simulink model "backbone"  (R2022b)
settings: Solver=FixedStepDiscrete  StartTime=0.0  StopTime=2  FixedStep=0.000001  RelTol=1e-3
undefined symbols (not defined in the file or in its folder): DiscIntNeverNeededParam, flux, Motor_flux, Motor_Ld_Indctances, Motor_Lq_Indctances, Motor_Pn, Motor_Rs, Pn, switch_electronic_feedworward, Switch_SubsysCtrl, SysCurrentMax, SysVoltage, Ts
libraries: powerlib_extras x11, simulink x4, mcbcontrolslib x4, slpidlib x3, spsPermanentMagnetSynchronousMachineLib x2, spsDCVoltageSourceLib x2, spsGroundLib x1, eePmsmCurrentController x1, spsThreePhaseVIMeasurementLib x1, spsTwoLevelConverterLib x1, spsUniversalBridgeLib x1, spspowerguiLib x1
(part 3 of 3)

== matlab function backbone/Variant Subsystem/MPTA_MPTV_PMSM/MPTA_弱磁/MPTA_MPTV_Base_IMax /MPTA_MPTV_Imax ==
  data: iqPIDref input; idref output; iqref output; UI input; LdLqPnFluxRs input; state output; clock input; we input; last_state input; We_A output; We_B output; Zone output; ctrl_way2 output; Te output
function [idref, iqref,state,We_A,We_B,Zone,ctrl_way2,Te] = fcn(iqPIDref, UI, LdLqPnFluxRs, clock, we, last_state)

% https://blog.csdn.net/weixin_44312889/article/details/124467496
%%%%%%%%%%%%%%%%%%%%%%%%%%%%%%%%%%%%%
%               读取数据
Udc=UI(1);
I=UI(2);
Ld=LdLqPnFluxRs(1);
Lq=LdLqPnFluxRs(2);
pn=LdLqPnFluxRs(3);%转子对数
flux=LdLqPnFluxRs(4);%永磁体磁链
R=LdLqPnFluxRs(5); %定子电阻
Zone=0;
ctrl_way2=0;

Umax=Udc/sqrt(3); %最大电压限制 此处应该是相电压最大值 
Imax=I*sqrt(2);% 最大电流限制

%%%%%%%%%%%%%%%%%%%%%%%%%%%%%%%%%%%%%
%               计算最大电流下MPTA与最大电流圆的交点A
IdA=(-flux+sqrt(flux^2+8*(Ld-Lq)^2*Imax^2))/(4*(Ld-Lq));
IqA=sqrt(Imax^2 - IdA^2);
We_A=sqrt(Umax^2/((Ld*IdA+flux)^2+(Lq*IqA)^2));
ctrl_way2=IqA;

%               计算最大电流下MPTV与最大电压圆的交点B
a=4*(Ld-Lq)^2*Ld^2+4*Lq^2*(Ld-Lq)^2;
b=8*flux*Ld*(Ld-Lq)^2+4*flux*Lq*(Ld-Lq)*Ld;
c=4*flux^2*(Ld-Lq)^2+4*flux^2*Lq*(Ld-Lq)-4*Lq^2*(Ld-Lq)^2*Imax^2;
IdB=(-b-sqrt(b^2-4*a*c))/(2*a);
tempB_a=-flux*Ld*(2*Ld-Lq);
tempB_b=2*(Ld^2+Lq^2)*(Ld-Lq);
tempB_c=Ld^2*(2*Ld-Lq)^2-4*Ld*(Ld-Lq)*(Ld^2+Lq^2);
tempB_d=Lq^2*(Ld-Lq)^2*(Ld^2+Lq^2);
tempB_e=sqrt(tempB_c*flux^2+4*Imax^2*tempB_d);

IdB=tempB_a+tempB_e/tempB_b;
IqB=sqrt(Imax^2-IdB^2);


We_B=sqrt(Umax^2/((Ld*IdB+flux)^2+(Lq*IqB)^2));
state=0;


% 进行MPTA控制 
iqref = iqPIDref;                           
idref=-flux+sqrt(flux^2+4*(Ld-Lq)^2*iqref^2)/(2*(Ld-Lq));

if(we<=We_A)
    if(iqPIDref<IqA) 
        % MPTA控制
        iqref = iqPIDref; % 此时进行MPTA控制   如果 iqref∈(-IqA,IqA)之间 则通过MPTA曲线上的idref
        idref=-flux+sqrt(flux^2+4*(Ld-Lq)^2*iqref^2)/(2*(Ld-Lq)); 
        Zone=0;
    else
        % 此时已达最大
        iqref=IqA;
        idref=IdA;
        Zone=1;
    end
elseif(we>We_A&&we<We_B)
       % FW iq id 沿着极限电压圆的轨迹变换
        idAB =(-flux*Ld+sqrt(flux^2*Ld^2-(Ld^2-Lq^2)*(flux^2+Lq^2*Imax^2-(Umax/we)^2)))/(Ld^2-Lq^2);
        iqAB =sqrt(Imax^2 - idAB^2);
        if(iqPIDref<iqAB)
            %idref=(-flux*Ld+sqrt(flux^2*Ld^2-(Ld^2-Lq^2)*(flux^2+Lq^2*iqPIDref^2-(Umax/we)^2)))/(Ld^2-Lq^2);
            temp=flux^2*Ld^2-(Ld^2-Lq^2)*(flux^2+Lq^2*iqPIDref^2-(Umax/we)^2); 
            idref=-(-flux*Ld+real(sqrt(complex(temp))))/(Ld^2-Lq^2);% 感觉我这步有点问题
            iqref=iqPIDref;
            Zone=2;
        else
            idref=idAB;
            iqref=iqAB;
            Zone=3;
        end
else %we > we_B MPTV
        idMTPV=-flux/Ld+(-flux*Lq+sqrt(flux^2*Lq^2+8*(Ld-Lq)^2*(Umax/we)^2))/(4*Ld*(Ld-Lq));
        iqMTPV=sqrt((Umax^2/we^2 - (Ld*idMTPV*flux)^2)/Lq^2); 
        if(iqPIDref<iqMTPV)
            iqref=iqPIDref;             
            idref=-flux/Ld+(-flux*Lq+Lq*sqrt(flux^2+4*(Ld-Lq)^2*iqref^2))/(2*Ld*(Ld-Lq));
            Zone=4;
        else
            idref=idMTPV;
            iqref=iqMTPV;
            Zone=5;
        end
end

        Te=3/2*pn*(flux*iqref+(Ld-Lq)*idref*iqref);
end

== matlab function backbone/Variant Subsystem/MPTA_MPTV_PMSM/MPTA_弱磁/MPTA_MPTV_Base_Te/MPTA_MPTV_Imax ==
  data: wx input; iqref_raw input; idref output; iqref output; UI input; LdLqPnFluxRs input; we input
function [idref, iqref] = fcn(wx,iqref_raw, UI, LdLqPnFluxRs, we)


%%%%%%%%%%%%%%%%%%%%%%%%%%%%%%%%%%%%%
%               读取数据


Udc=UI(1);
I=UI(2);
Ld=LdLqPnFluxRs(1);
Lq=LdLqPnFluxRs(2);
pn=LdLqPnFluxRs(3);
flux=LdLqPnFluxRs(4);
R=LdLqPnFluxRs(5);
psif=flux;

Umax=Udc*2/pi;
Imax=I*sqrt(2);

%%%%%%%%%%%%%%%%%%%%%%%%%%%%%%%%%%%%%

% id=0;
% iq=0;
p=Lq/Ld;%凸极率
num = flux^2+8*(Ld-Lq)^2*Ilim^2;
C = -flux+sqrt(num);
num0 = (Lq*Ilim)^2+flux^2+((Ld+Lq)*C^2+8*flux*Ld*C)/(16*(Ld-Lq));
nb = 60*Ulim/(2*pi*sqrt(num0));
wb = Pn*nb*pi/30;%基速 电角速度
% id、iq是电流环的给定，也就是MTPA的输出，无法用星号表示
% MPTA相关
    num1 = 8*Te*flux/(3*Pn);
    num2 = flux^2-4*(Ld-Lq)^2;
    num4 = num1^2-4*num2*((0.5*num1/flux)^2-flux^2);
    
    num3 = flux*0.5/(Lq-Ld);
    
    
if(wx<=wb)                % MPTA
    % 第一步 计算iq
    iq = (num1+sqrt(num4))/(2*num2);
 
    %第二步 计算id
    num5 = 0.25*flux^2/(Ld-Lq)^2+iq^2;
    id = num3-sqrt(num5);
else                      %弱磁控制
    if(we<wx)      %到达C点之前       
        if(flux/Ld>Ilim)
            num6 = flux^2*Ld^2-(Ld^2-Lq^2)*(flux^2-Ulim^2/wx^2+Lq^2*Ilim^2);
            id = (-flux*Ld+sqrt(num6))/(Ld^2-Lq^2);
            num7 = Ilim^2-id^2;
            iq = sqrt(num7); %显 示7为负
        else
            num8 = flux^2*Ld^2-(Lq^2-Ld^2)*(Ulim^2/wx^2 - flux^2 - Lq^2*Ilim^2);
            id = (flux*Ld-sqrt(num8))/(Ld^2-Lq^2);  
            num7 = Ilim^2-id^2;
            iq = sqrt(num7); %显示7为负
        end
    else                %到达C点后
        if(flux/Ld>Ilim)
            iq = (num1+sqrt(num4))/(2*num2);
            num9 = (Ulim/(Ld*wx))^2-(p*iq)^2;
            id = -flux/Ld+sqrt(num9);
        else
            iq = (num1+sqrt(num4))/(2*num2);
            num9 = (Ulim/(Ld*wx))^2-(p*iq)^2;
            id = -flux/Ld-sqrt(num9);    
        end
    end
end 
end

== matlab function backbone/Variant Subsystem/MPTA_MPTV_PMSM/MPTA_弱磁/MPTA_MPTV_Base_IMax /MPTA_MPTV_Imax1 ==
  data: iqPIDref input; idref output; iqref output; UI input; LdLqPnFluxRs input; state output; clock input; we input; last_state input; we_A output; we_B output; ctrl_way output; ctrl_way2 output; Te output
function [idref, iqref,state,we_A,we_B,ctrl_way,ctrl_way2,Te] = fcn(iqPIDref, UI, LdLqPnFluxRs, clock, we, last_state)

% https://blog.csdn.net/weixin_44312889/article/details/124467496
%%%%%%%%%%%%%%%%%%%%%%%%%%%%%%%%%%%%%
%               读取数据
Udc=UI(1);
I=UI(2);
Ld=LdLqPnFluxRs(1);
Lq=LdLqPnFluxRs(2);
pn=LdLqPnFluxRs(3);%转子对数
flux=LdLqPnFluxRs(4);%永磁体磁链
R=LdLqPnFluxRs(5); %定子电阻
psif=flux;% 
ctrl_way=0;
ctrl_way2=0;

Umax=Udc/sqrt(3); %最大电压限制 此处应该是相电压最大值 
Imax=I*sqrt(2);% 最大电流限制

%%%%%%%%%%%%%%%%%%%%%%%%%%%%%%%%%%%%%
%               计算最大电流下MPTA与最大电流圆的交点A
IdA=(-psif+sqrt(psif^2+8*(Ld-Lq)^2*Imax^2))/(4*(Ld-Lq));
IqA=sqrt(Imax^2 - IdA^2);
we_A=sqrt(Umax^2/((Ld*IdA+psif)^2+(Lq*IqA)^2));


%               计算最大电流下MPTV与最大电压圆的交点B
a=4*(Ld-Lq)^2*Ld^2+4*Lq^2*(Ld-Lq)^2;
b=8*psif*Ld*(Ld-Lq)^2+4*psif*Lq*(Ld-Lq)*Ld;
c=4*psif^2*(Ld-Lq)^2+4*psif^2*Lq*(Ld-Lq)-4*Lq^2*(Ld-Lq)^2*Imax^2;
IdB=(-b-sqrt(b^2-4*a*c))/(2*a);
tempB_a=-psif*Ld*(2*Ld-Lq);
tempB_b=2*(Ld^2+Lq^2)*(Ld-Lq);
tempB_c=Ld^2*(2*Ld-Lq)^2-4*Ld*(Ld-Lq)*(Ld^2+Lq^2);
tempB_d=Lq^2*(Ld-Lq)^2*(Ld^2+Lq^2);
tempB_e=sqrt(tempB_c*psif^2+4*Imax^2*tempB_d);

IdB=tempB_a+tempB_e/tempB_b;
IqB=sqrt(Imax^2-IdB^2);


we_B=sqrt(Umax^2/((Ld*IdB+psif)^2+(Lq*IqB)^2));


%%%%%%%%%%%%%%%%%%%%%%%%%%%%%%%%%%%%%
% 状态切换
if(clock==0)
    last_state=1; 
end

state=last_state;

% 定义有限状态机
switch state
    case 1
        if(iqPIDref >= IqA)                            % 将iq id 界定在极限电流源以内
            iqref=IqA;
            idref=IdA;  
        elseif(iqPIDref <= -IqA)
            iqref=-IqA;
            idref=IdA;
        else
            iqref = iqPIDref;                           % 此时进行MPTA控制   如果 iqref∈(-IqA,IqA)之间 则通过MPTA曲线上的idref
            idref=-psif+sqrt(psif^2+4*(Ld-Lq)^2*iqref^2)/(2*(Ld-Lq)); 
            ctrl_way=1;
        end

        if(abs(we)>we_A)                                % 在电机开始转动速率开始爬升时，一旦we突破了we_A界限 就得通过弱磁控制+MPTA的方式去输出idref和iqref 
            state=2;
            ctrl_way=2;
        end

    otherwise
        % 这一部分是 为了计算出当前速度所对应的iq值 其实就是clark-park变换所得到的当前旋转坐标轴下的定子电流iq id
        if(abs(we)<=we_A)                               % 当输出转速小于该转矩下的最小转速时，iq限制电流等于iqA 
            iqCur=IqA;
            ctrl_way2=3;
        elseif( abs(we)>=we_A && abs(we)<=we_B )        % 当速度小于we_A<we<we_B 则通过电压极限圆和电流极限圆的交点所得的id iq为限制条件 沿着AB段
            idCur =(-psif*Ld+sqrt(psif^2*Ld^2-(Ld^2-Lq^2)*(psif^2+Lq^2*Imax^2-(Umax/we)^2)))/(Ld^2-Lq^2);
            iqCur =sqrt(Imax^2 - idCur^2);
            ctrl_way2=4;            
        else                                            %we>we_B 则通过MTPV曲线公式去推导出idlim和iqCur  
            %Ldid_psif=(-psif*Lq+sqrt(psif^2*Lq^2+8*(Ld-Lq)^2*(Umax/we)^2))/(4*(Ld-Lq));
            %idCur=(Ldid_psif-psif)/Ld;
            idCur=-psif/Ld+(-psif*Lq+sqrt(psif^2*Lq^2+8*(Ld-Lq)^2*(Umax/we)^2))/(4*Ld*(Ld-Lq));
            iqCur=sqrt((Umax^2/we^2 - (Ld*idCur*psif)^2)/Lq^2);
            ctrl_way2=5;            
        end
        
        %%
        % 接下来if 和 elseif的目的是一个意思 要让电流运动在极限电压源和极限电流源的范围内 一个是第二象限 一个是第四象限的判断
        % 只分析第一个if 由于该仿真假设了前提条件:速度只增加 不减小
        % 当通过PI控制输出的iqRef丹玉iqCur时，通过等转矩曲线我们可以知道，此时的速度实际上是降低的
        % 根据前提条件速度只增加，不减小。故进入此判断
        % 第二个if是指，当iqCur>IqB说明此时还正处于弱磁I区，弱磁一区中iq ir的变化趋势就等同于在Imax的极限电流圆上跑
        % 同理紧接着的else，iqCur<IqB就是指当前已处于MPTV区，弱磁一区中iq ir的变化趋势就等同于在Imax的MPTV曲线上跑
        % 
        % 疑问点：为何不将iqref=iqCur idref=idCur 而是将idref又重新计算了一遍
        % 1：通过we去判断当前处于哪一个区间，并基于那个区间的控制方式和we与iq id的耦合关系，求出此时的id iq 
        % 2：不难过看出此时的id iq不仅仅可以用上面的公式求出，还可以通过clark-park变换求出
        % 3：所以上面除了if(abs(we)<=we_A)的，其他两个判断可以不用做。只需要将clark-park变换得到的iq id
        %   等于对应的idCur iqCur即可。
        %%
        if(iqPIDref > min(iqCur,IqA)) 
            if(min(iqCur,IqA)>IqB)
                idref = -sqrt(Imax^2 - min(iqCur,IqA)^2);
                iqref = min(iqCur,IqA);
                ctrl_way=6;                
            else
                ctrl_way=7;     
                idref=-psif/Ld+(-psif*Lq+Lq*sqrt(psif^2+4*(Ld-Lq)^2*iqCur^2))/(2*Ld*(Ld-Lq)); %MPTV
                iqref=iqCur;
            end
        elseif(iqPIDref < max(-iqCur,-IqA))
            if(max(-iqCur,-IqA) < -IqB)
                ctrl_way=8;                     
                idref = -sqrt(Imax^2 - max(-iqCur,-IqA)^2);
                iqref = max(-iqCur,-IqA);                  
            else
                ctrl_way=9;     
                idref=-psif/Ld+(-psif*Lq+Lq*sqrt(psif^2+4*(Ld-Lq)^2*iqCur^2))/(2*Ld*(Ld-Lq));%MPTV
                iqref=iqCur;
            end
        else    
            if(iqPIDref > IqB)%弱磁控制 沿着AB段运动
                %FW
                ctrl_way=10;
                idref = -sqrt(Imax^2 -iqPIDref^2);
                iqref = iqPIDref;
            elseif(iqPIDref<IqB && iqPIDref > -IqB) % 沿着MPTV曲线运动 BC段
                %MPTV
                ctrl_way=11;
                idref=-psif/Ld+(-psif*Lq+Lq*sqrt(psif^2+4*(Ld-Lq)^2*iqPIDref^2))/(2*Ld*(Ld-Lq));%MPTV
                iqref=iqPIDref;   
            else% 弱磁控制 沿着AB段运动
                %FW
                 ctrl_way=12;
                idref = -sqrt(Imax^2 -iqPIDref^2);
                iqref = iqPIDref;
            end
        end
end
Te=3/2*pn*(flux*iqref+(Ld-Lq)*idref*iqref);

end
